simulink library "radar_switch_lib"  (Simulink 8.2)
settings: Solver=ode1  StartTime=0.0  StopTime=Inf  FixedStep=0.001  RelTol=1e-3
PostLoadFcn:
  | , if any(exist('dsrtsu_mdlpostloadfcn', 'file') == [2, 3, 6]), try dsrtsu_mdlpostloadfcn('Execute', bdroot); catch fprintf('Error in PostLoadFcn (dsrtsu_mdlpostloadfcn) for model "%s":\n %s\n', bdroot, lasterr); end, end,
libraries: simulink x4
settings Model: DSRTSU_INTERNAL_RTI_VER=450  DSRTSU_INTERNAL_RTI_TYPE=rti1401  DSRTSU_INTERNAL_RTIFPGA=40  Creator=rushk1  LastModifiedBy=rushk1

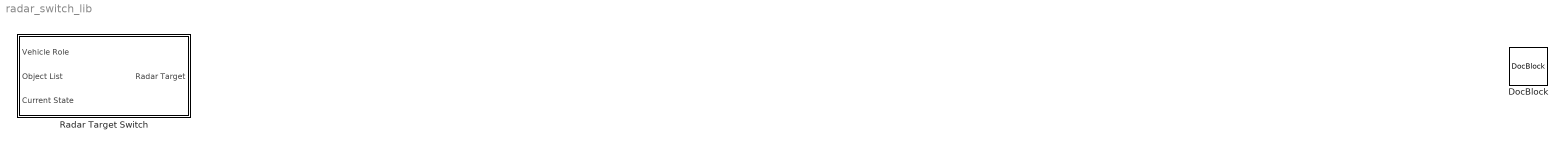
== system radar_switch_lib ==
  DocBlock : simulink/Model-Wide Utilities/DocBlock  DocumentType=Text
      content=|
      | This library is responsible for handling radar target selection.
      |
      | The radar target of the follow vehicle in particular is subject to change
      | throughout the course of a run. Initially, the follow vehicle targets the
      | second (in the event it can also see the merge vehicle) or first (in the
      | case it can only see one object) object it can see. The intent is that it
      | should follow the lead vehicle as it's target. Upon attaining merge ready
      | and from thereafter it changes target to the closest object, the merge
      | vehicle.
      |
      | The merge vehicle always follows the closest object as its radar target.
  Radar Target Switch : Subsystem

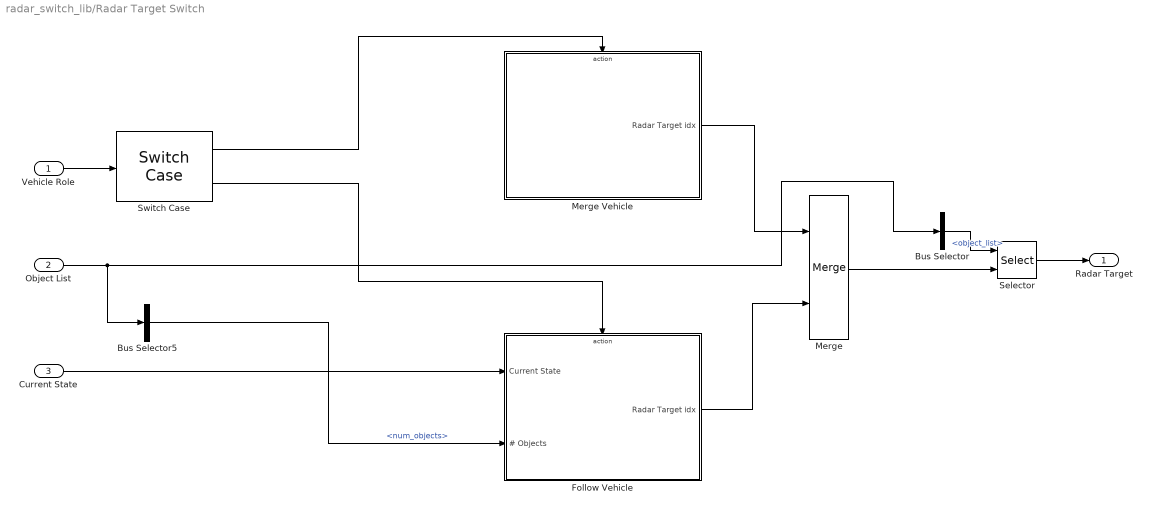
== system radar_switch_lib/Radar Target Switch ==
  Vehicle Role : Inport
  Object List : Inport  Port=2  OutDataTypeStr=Bus: DetailedObjectList
  Current State : Inport  Port=3
  Bus Selector : BusSelector  OutputSignals=object_list
  Bus Selector5 : BusSelector  OutputSignals=num_objects
  Follow Vehicle : Subsystem  TreatAsAtomicUnit=on
  Merge : Merge
  Merge Vehicle : Subsystem  TreatAsAtomicUnit=on
  Selector : Selector  InputPortWidth=4  IndexOptions=Index vector (port)  Indices=[1 3]  OutputSizes=1
  Switch Case : SwitchCase  CaseConditions={VehicleRoleEnum.MERGE, VehicleRoleEnum.FOLLOW}  ShowDefaultCase=off
  Radar Target : Outport  OutDataTypeStr=Bus: FusObjectTrackA
  wires:
  Vehicle Role/1 -> Switch Case/1
  Switch Case/1 -> Merge Vehicle/Action
  Switch Case/2 -> Follow Vehicle/Action
  Current State/1 -> Follow Vehicle/1(Current State)
  Follow Vehicle/1(Radar Target idx) -> Merge/2
  Merge Vehicle/1(Radar Target idx) -> Merge/1
  Merge/1 -> Selector/2
  Bus Selector/1 -> Selector/1  "<object_list>"
  Selector/1 -> Radar Target/1
  Object List/1 -> Bus Selector5/1, Bus Selector/1
  Bus Selector5/1 -> Follow Vehicle/2(# Objects)  "<num_objects>"

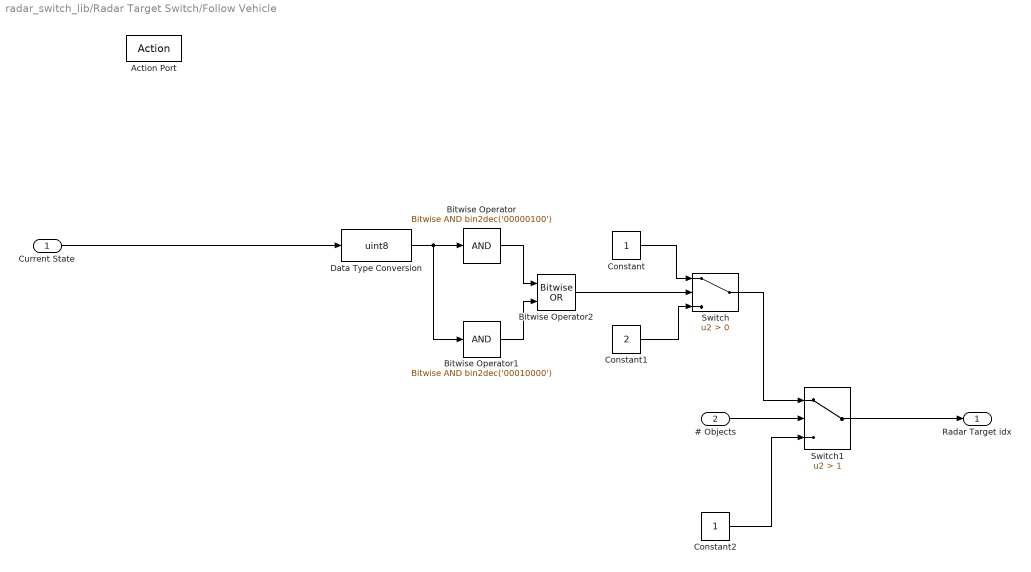
== system radar_switch_lib/Radar Target Switch/Follow Vehicle ==
  Current State : Inport
  # Objects : Inport  Port=2
  Action Port : ActionPort  ActionType=case
  Bitwise Operator : simulink/Logic and Bit Operations/Bitwise Operator  logicop=AND  UseBitMask=on  BitMask=bin2dec('00000100')  BitMaskRealWorld=Stored Integer
  Bitwise Operator1 : simulink/Logic and Bit Operations/Bitwise Operator  logicop=AND  UseBitMask=on  BitMask=bin2dec('00010000')  BitMaskRealWorld=Stored Integer
  Bitwise Operator2 : simulink/Logic and Bit Operations/Bitwise Operator  logicop=OR  UseBitMask=off  NumInputPorts=2  BitMask=bin2dec('11011001')  BitMaskRealWorld=Stored Integer
  Constant : Constant
  Constant1 : Constant  Value=2
  Constant2 : Constant
  Data Type Conversion : DataTypeConversion  OutDataTypeStr=uint8
  Switch : Switch  Criteria=u2 > Threshold
  Switch1 : Switch  Criteria=u2 > Threshold  Threshold=1
  Radar Target idx : Outport
  wires:
  Current State/1 -> Data Type Conversion/1
  Data Type Conversion/1 -> Bitwise Operator/1, Bitwise Operator1/1
  Bitwise Operator2/1 -> Switch/2
  Bitwise Operator/1 -> Bitwise Operator2/1
  Bitwise Operator1/1 -> Bitwise Operator2/2
  Constant/1 -> Switch/1
  Constant1/1 -> Switch/3
  Switch/1 -> Switch1/1
  # Objects/1 -> Switch1/2
  Switch1/1 -> Radar Target idx/1
  Constant2/1 -> Switch1/3

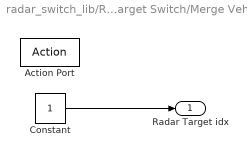
== system radar_switch_lib/Radar Target Switch/Merge Vehicle ==
  Action Port : ActionPort  ActionType=case
  Constant : Constant
  Radar Target idx : Outport
  wires:
  Constant/1 -> Radar Target idx/1
